simulink model "TS"  (R2024a)
settings: Solver=VariableStepAuto  StartTime=0.0  StopTime=10*10^-6  RelTol=1e-3
undefined symbols (not defined in the file): c1, c3
libraries: commblkcod2 x1, commofdm x1, commdigbbndam3 x1, commseqgen3 x1
settings Model: Creator=Honest  LastModifiedBy=NEYMAR
settings RTWCC: GPUComputeCapability=3.5

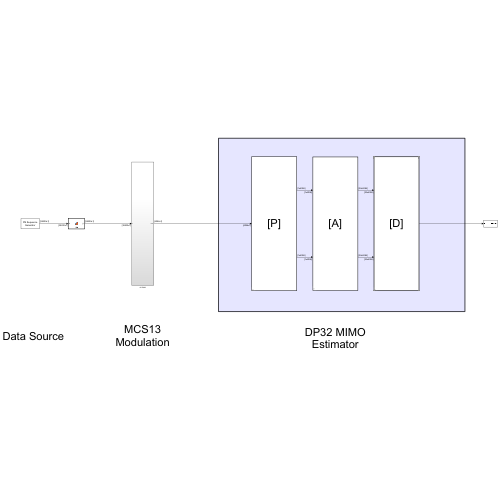
[thumbnail: Simulink's stored preview of the top-level diagram]
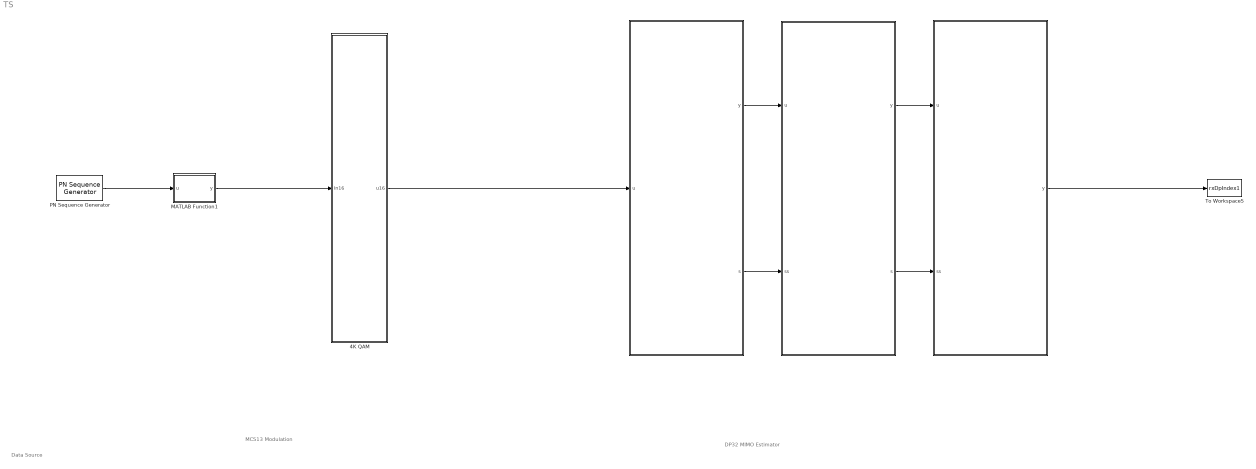
== system TS ==
  note: Data Source
  note: MCS13 Modulation
  note: DP32 MIMO Estimator
  " " : MATLAB Function  TreatAsAtomicUnit=on
  " " : MATLAB Function  TreatAsAtomicUnit=on
  "    " : MATLAB Function  TreatAsAtomicUnit=on
  4K QAM : Subsystem
  MATLAB Function1 : MATLAB Function  TreatAsAtomicUnit=on
  PN Sequence Generator : commseqgen3/PN Sequence Generator  poly='z^15 + z^14 + 1'  ini_sta=[0 0 0 0 0 0 0 0 0 0 0 0 0 0 1]  outBitMaskSource=Dialog parameter  shift=0  outVarSiz=off  maxOutSizeMode=Dialog parameter  maxOutSize=[10 1]  Ts=3.472222*10^-10  sampPerFrame=39200  reset=off  bitPackedOutputs=off  outDataType=double  numPackedBits=8  bitPackDataSigned=off  bitPackedOutDType=double
  To Workspace5 : ToWorkspace  VariableName=rxDpIndex1  SampleTime=-1
      settings: MaxDataPoints=1  Save2DSignal=2-D array (concatenate along first dimension)
  wires:
  4K QAM/1(u16) -> " "/1(u)
  PN Sequence Generator/1 -> MATLAB Function1/1(u)
  " "/1(y) -> "    "/1(u)
  "    "/1(y) -> " "/1(u)
  " "/1(y) -> To Workspace5/1
  " "/2(s) -> "    "/2(ss)
  "    "/2(s) -> " "/2(ss)
  MATLAB Function1/1(y) -> 4K QAM/1(In16)

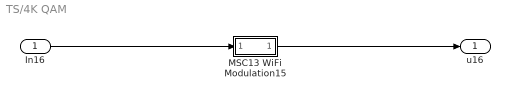
== system TS/4K QAM ==
  In16 : Inport
  MSC13 WiFi Modulation15 : Subsystem
  u16 : Outport
  wires:
  In16/1 -> MSC13 WiFi Modulation15/1(In1)
  MSC13 WiFi Modulation15/1(Out1) -> u16/1

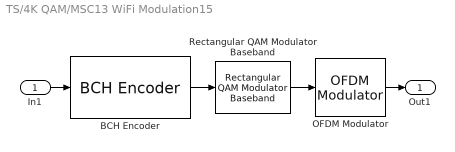
== system TS/4K QAM/MSC13 WiFi Modulation15 ==
  In1 : Inport
  BCH Encoder : commblkcod2/BCH Encoder  n=47040  k=39200  specShortening=off  shortenedK=5  specGenPoly=off  genPoly='X^10 + X^8 + X^5 + X^4 + X^2 + X + 1'  specPrimPoly=off  prPoly='X^4 + X + 1'  specDisableGenCheck=off  specPuncture=off  punctVec=[ones(8,1); zeros(2,1)]
  OFDM Modulator : commofdm/OFDM Modulator  StatePerturbationForJacobian=1.0e-05  FFTLength=4096  NumGuardBandCarriers=[88; 88]  InsertDCNull=off  PilotInputPort=off  PilotCarrierIndices=[52;104;156;208;260]  CyclicPrefixLength=0  Windowing=off  WindowLength=1  OversamplingFactor=1  NumSymbols=1  NumTransmitAntennas=1  SimulateUsing=Interpreted execution
  Rectangular QAM Modulator Baseband : commdigbbndam3/Rectangular QAM Modulator Baseband  M=4096  InType=Bit  Enc=Gray  Mapping=[0:15]  PowType=Min. distance between symbols  MinDist=2  AvgPow=1  PeakPow=1  Ph=0  outDtype=double  outWordLen=16  outUDDataType=sfix(16)  outFracLenMode=Best precision  outFracLen=15  outDataTypeStr=double  outLastDataTypeStr=double
  Out1 : Outport
  wires:
  Rectangular QAM Modulator Baseband/1 -> OFDM Modulator/1
  OFDM Modulator/1 -> Out1/1
  BCH Encoder/1 -> Rectangular QAM Modulator Baseband/1
  In1/1 -> BCH Encoder/1

== matlab function TS/MATLAB Function1 ==
  data: u input; y output
function y = fcn(u)

u(1:39200,1) = 1;

y = u;

== matlab function TS/  ==
  data: u input; y output; s output
function [y, s] = fcn(u)
    
        Walsh = [
            1	1	1	1	1	1	1	1	1	1	1	1	1	1	1	1	1	1	1	1	1	1	1	1	1	1	1	1	1	1	1	1;
																															    
            1	-1	1	-1	1	-1	1	-1	1	-1	1	-1	1	-1	1	-1	1	-1	1	-1	1	-1	1	-1	1	-1	1	-1	1	-1	1	-1;
																															            
            1	1	-1	-1	1	1	-1	-1	1	1	-1	-1	1	1	-1	-1	1	1	-1	-1	1	1	-1	-1	1	1	-1	-1	1	1	-1	-1;
																															            
            1	-1	-1	1	1	-1	-1	1	1	-1	-1	1	1	-1	-1	1	1	-1	-1	1	1	-1	-1	1	1	-1	-1	1	1	-1	-1	1;
																															            
            1	1	1	1	-1	-1	-1	-1	1	1	1	1	-1	-1	-1	-1	1	1	1	1	-1	-1	-1	-1	1	1	1	1	-1	-1	-1	-1;
																															            
            1	-1	1	-1	-1	1	-1	1	1	-1	1	-1	-1	1	-1	1	1	-1	1	-1	-1	1	-1	1	1	-1	1	-1	-1	1	-1	1;
																															            
            1	1	-1	-1	-1	-1	1	1	1	1	-1	-1	-1	-1	1	1	1	1	-1	-1	-1	-1	1	1	1	1	-1	-1	-1	-1	1	1;
																															            
            1	-1	-1	1	-1	1	1	-1	1	-1	-1	1	-1	1	1	-1	1	-1	-1	1	-1	1	1	-1	1	-1	-1	1	-1	1	1	-1;
																															            
            1	1	1	1	1	1	1	1	-1	-1	-1	-1	-1	-1	-1	-1	1	1	1	1	1	1	1	1	-1	-1	-1	-1	-1	-1	-1	-1;
																															            
            1	-1	1	-1	1	-1	1	-1	-1	1	-1	1	-1	1	-1	1	1	-1	1	-1	1	-1	1	-1	-1	1	-1	1	-1	1	-1	1;
																															            
            1	1	-1	-1	1	1	-1	-1	-1	-1	1	1	-1	-1	1	1	1	1	-1	-1	1	1	-1	-1	-1	-1	1	1	-1	-1	1	1;
																															            
            1	-1	-1	1	1	-1	-1	1	-1	1	1	-1	-1	1	1	-1	1	-1	-1	1	1	-1	-1	1	-1	1	1	-1	-1	1	1	-1;
																															            
            1	1	1	1	-1	-1	-1	-1	-1	-1	-1	-1	1	1	1	1	1	1	1	1	-1	-1	-1	-1	-1	-1	-1	-1	1	1	1	1;
																															            
            1	-1	1	-1	-1	1	-1	1	-1	1	-1	1	1	-1	1	-1	1	-1	1	-1	-1	1	-1	1	-1	1	-1	1	1	-1	1	-1;
																															            
            1	1	-1	-1	-1	-1	1	1	-1	-1	1	1	1	1	-1	-1	1	1	-1	-1	-1	-1	1	1	-1	-1	1	1	1	1	-1	-1;
																															            
            1	-1	-1	1	-1	1	1	-1	-1	1	1	-1	1	-1	-1	1	1	-1	-1	1	-1	1	1	-1	-1	1	1	-1	1	-1	-1	1;
																															            
            1	1	1	1	1	1	1	1	1	1	1	1	1	1	1	1	-1	-1	-1	-1	-1	-1	-1	-1	-1	-1	-1	-1	-1	-1	-1	-1;
																															            
            1	-1	1	-1	1	-1	1	-1	1	-1	1	-1	1	-1	1	-1	-1	1	-1	1	-1	1	-1	1	-1	1	-1	1	-1	1	-1	1;
																															            
            1	1	-1	-1	1	1	-1	-1	1	1	-1	-1	1	1	-1	-1	-1	-1	1	1	-1	-1	1	1	-1	-1	1	1	-1	-1	1	1;
																															            
            1	-1	-1	1	1	-1	-1	1	1	-1	-1	1	1	-1	-1	1	-1	1	1	-1	-1	1	1	-1	-1	1	1	-1	-1	1	1	-1;
																															            
            1	1	1	1	-1	-1	-1	-1	1	1	1	1	-1	-1	-1	-1	-1	-1	-1	-1	1	1	1	1	-1	-1	-1	-1	1	1	1	1;
																															            
            1	-1	1	-1	-1	1	-1	1	1	-1	1	-1	-1	1	-1	1	-1	1	-1	1	1	-1	1	-1	-1	1	-1	1	1	-1	1	-1;
																															            
            1	1	-1	-1	-1	-1	1	1	1	1	-1	-1	-1	-1	1	1	-1	-1	1	1	1	1	-1	-1	-1	-1	1	1	1	1	-1	-1;
																															            
            1	-1	-1	1	-1	1	1	-1	1	-1	-1	1	-1	1	1	-1	-1	1	1	-1	1	-1	-1	1	-1	1	1	-1	1	-1	-1	1;
																															            
            1	1	1	1	1	1	1	1	-1	-1	-1	-1	-1	-1	-1	-1	-1	-1	-1	-1	-1	-1	-1	-1	1	1	1	1	1	1	1	1;
																															            
            1	-1	1	-1	1	-1	1	-1	-1	1	-1	1	-1	1	-1	1	-1	1	-1	1	-1	1	-1	1	1	-1	1	-1	1	-1	1	-1;
																															            
            1	1	-1	-1	1	1	-1	-1	-1	-1	1	1	-1	-1	1	1	-1	-1	1	1	-1	-1	1	1	1	1	-1	-1	1	1	-1	-1;
																															            
            1	-1	-1	1	1	-1	-1	1	-1	1	1	-1	-1	1	1	-1	-1	1	1	-1	-1	1	1	-1	1	-1	-1	1	1	-1	-1	1;
																															            
            1	1	1	1	-1	-1	-1	-1	-1	-1	-1	-1	1	1	1	1	-1	-1	-1	-1	1	1	1	1	1	1	1	1	-1	-1	-1	-1;
																															            
            1	-1	1	-1	-1	1	-1	1	-1	1	-1	1	1	-1	1	-1	-1	1	-1	1	1	-1	1	-1	1	-1	1	-1	-1	1	-1	1;
																															            
            1	1	-1	-1	-1	-1	1	1	-1	-1	1	1	1	1	-1	-1	-1	-1	1	1	1	1	-1	-1	1	1	-1	-1	-1	-1	1	1;
																															            
            1	-1	-1	1	-1	1	1	-1	-1	1	1	-1	1	-1	-1	1	-1	1	1	-1	1	-1	-1	1	1	-1	-1	1	-1	1	1	-1;
        ];

        Increased_Walsh = Walsh(:, repelem(1:size(Walsh, 2), 16));
        
        Ext_Walsh = repmat(Increased_Walsh, [1, 8]);
        
        % 32 streams
        ProcessedInput = reshape(u,4096,1)';
        
        % Polarization
        Polarization = Ext_Walsh(1, :);
        assignin('base', "P", Polarization);

y = Polarization;
s = ProcessedInput;

== matlab function TS/     ==
  data: u input; y output; ss input; s output
function [y, s] = fcn(u, ss)

        % Aggregated polarization
        TempAggregatedPolarization = reshape(u', 1, []);
        TAPRowClone = repmat(TempAggregatedPolarization, 32, 1);
        assignin('base', 'PA', TAPRowClone);

        % Aggregated streams
        TempAggregatedProcessedInput = reshape(ss, 1, 4096);
        TAPIRowClone = repmat(TempAggregatedProcessedInput, 32, 1);
        
y = TAPRowClone;
s = TAPIRowClone;

== matlab function TS/  ==
  data: u input; y output; ss input; c1 parameter; c3 parameter
function y = fcn(u, ss, c1, c3)
        
        Walsh = [
            1	1	1	1	1	1	1	1	1	1	1	1	1	1	1	1	1	1	1	1	1	1	1	1	1	1	1	1	1	1	1	1;
																															    
            1	-1	1	-1	1	-1	1	-1	1	-1	1	-1	1	-1	1	-1	1	-1	1	-1	1	-1	1	-1	1	-1	1	-1	1	-1	1	-1;
																															            
            1	1	-1	-1	1	1	-1	-1	1	1	-1	-1	1	1	-1	-1	1	1	-1	-1	1	1	-1	-1	1	1	-1	-1	1	1	-1	-1;
																															            
            1	-1	-1	1	1	-1	-1	1	1	-1	-1	1	1	-1	-1	1	1	-1	-1	1	1	-1	-1	1	1	-1	-1	1	1	-1	-1	1;
																															            
            1	1	1	1	-1	-1	-1	-1	1	1	1	1	-1	-1	-1	-1	1	1	1	1	-1	-1	-1	-1	1	1	1	1	-1	-1	-1	-1;
																															            
            1	-1	1	-1	-1	1	-1	1	1	-1	1	-1	-1	1	-1	1	1	-1	1	-1	-1	1	-1	1	1	-1	1	-1	-1	1	-1	1;
																															            
            1	1	-1	-1	-1	-1	1	1	1	1	-1	-1	-1	-1	1	1	1	1	-1	-1	-1	-1	1	1	1	1	-1	-1	-1	-1	1	1;
																															            
            1	-1	-1	1	-1	1	1	-1	1	-1	-1	1	-1	1	1	-1	1	-1	-1	1	-1	1	1	-1	1	-1	-1	1	-1	1	1	-1;
																															            
            1	1	1	1	1	1	1	1	-1	-1	-1	-1	-1	-1	-1	-1	1	1	1	1	1	1	1	1	-1	-1	-1	-1	-1	-1	-1	-1;
																															            
            1	-1	1	-1	1	-1	1	-1	-1	1	-1	1	-1	1	-1	1	1	-1	1	-1	1	-1	1	-1	-1	1	-1	1	-1	1	-1	1;
																															            
            1	1	-1	-1	1	1	-1	-1	-1	-1	1	1	-1	-1	1	1	1	1	-1	-1	1	1	-1	-1	-1	-1	1	1	-1	-1	1	1;
																															            
            1	-1	-1	1	1	-1	-1	1	-1	1	1	-1	-1	1	1	-1	1	-1	-1	1	1	-1	-1	1	-1	1	1	-1	-1	1	1	-1;
																															            
            1	1	1	1	-1	-1	-1	-1	-1	-1	-1	-1	1	1	1	1	1	1	1	1	-1	-1	-1	-1	-1	-1	-1	-1	1	1	1	1;
																															            
            1	-1	1	-1	-1	1	-1	1	-1	1	-1	1	1	-1	1	-1	1	-1	1	-1	-1	1	-1	1	-1	1	-1	1	1	-1	1	-1;
																															            
            1	1	-1	-1	-1	-1	1	1	-1	-1	1	1	1	1	-1	-1	1	1	-1	-1	-1	-1	1	1	-1	-1	1	1	1	1	-1	-1;
																															            
            1	-1	-1	1	-1	1	1	-1	-1	1	1	-1	1	-1	-1	1	1	-1	-1	1	-1	1	1	-1	-1	1	1	-1	1	-1	-1	1;
																															            
            1	1	1	1	1	1	1	1	1	1	1	1	1	1	1	1	-1	-1	-1	-1	-1	-1	-1	-1	-1	-1	-1	-1	-1	-1	-1	-1;
																															            
            1	-1	1	-1	1	-1	1	-1	1	-1	1	-1	1	-1	1	-1	-1	1	-1	1	-1	1	-1	1	-1	1	-1	1	-1	1	-1	1;
																															            
            1	1	-1	-1	1	1	-1	-1	1	1	-1	-1	1	1	-1	-1	-1	-1	1	1	-1	-1	1	1	-1	-1	1	1	-1	-1	1	1;
																															            
            1	-1	-1	1	1	-1	-1	1	1	-1	-1	1	1	-1	-1	1	-1	1	1	-1	-1	1	1	-1	-1	1	1	-1	-1	1	1	-1;
																															            
            1	1	1	1	-1	-1	-1	-1	1	1	1	1	-1	-1	-1	-1	-1	-1	-1	-1	1	1	1	1	-1	-1	-1	-1	1	1	1	1;
																															            
            1	-1	1	-1	-1	1	-1	1	1	-1	1	-1	-1	1	-1	1	-1	1	-1	1	1	-1	1	-1	-1	1	-1	1	1	-1	1	-1;
																															            
            1	1	-1	-1	-1	-1	1	1	1	1	-1	-1	-1	-1	1	1	-1	-1	1	1	1	1	-1	-1	-1	-1	1	1	1	1	-1	-1;
																															            
            1	-1	-1	1	-1	1	1	-1	1	-1	-1	1	-1	1	1	-1	-1	1	1	-1	1	-1	-1	1	-1	1	1	-1	1	-1	-1	1;
																															            
            1	1	1	1	1	1	1	1	-1	-1	-1	-1	-1	-1	-1	-1	-1	-1	-1	-1	-1	-1	-1	-1	1	1	1	1	1	1	1	1;
																															            
            1	-1	1	-1	1	-1	1	-1	-1	1	-1	1	-1	1	-1	1	-1	1	-1	1	-1	1	-1	1	1	-1	1	-1	1	-1	1	-1;
																															            
            1	1	-1	-1	1	1	-1	-1	-1	-1	1	1	-1	-1	1	1	-1	-1	1	1	-1	-1	1	1	1	1	-1	-1	1	1	-1	-1;
																															            
            1	-1	-1	1	1	-1	-1	1	-1	1	1	-1	-1	1	1	-1	-1	1	1	-1	-1	1	1	-1	1	-1	-1	1	1	-1	-1	1;
																															            
            1	1	1	1	-1	-1	-1	-1	-1	-1	-1	-1	1	1	1	1	-1	-1	-1	-1	1	1	1	1	1	1	1	1	-1	-1	-1	-1;
																															            
            1	-1	1	-1	-1	1	-1	1	-1	1	-1	1	1	-1	1	-1	-1	1	-1	1	1	-1	1	-1	1	-1	1	-1	-1	1	-1	1;
																															            
            1	1	-1	-1	-1	-1	1	1	-1	-1	1	1	1	1	-1	-1	-1	-1	1	1	1	1	-1	-1	1	1	-1	-1	-1	-1	1	1;
																															            
            1	-1	-1	1	-1	1	1	-1	-1	1	1	-1	1	-1	-1	1	-1	1	1	-1	1	-1	-1	1	1	-1	-1	1	-1	1	1	-1;
        ];

        Increased_Walsh = Walsh(:, repelem(1:size(Walsh, 2), 16));
        
        Ext_Walsh = repmat(Increased_Walsh, [1, 8]);
        
        % Polarization to be multiplied to Receieved Polarization
        R_matrix = Ext_Walsh;
        
        % Multiplication of Polarization and Depolarization
        Result_matrix = u .* R_matrix;
        assignin('base', 'PAD', Result_matrix);
        
        % Sample by sample, Replace 1s with cos, -1s with sin
        % c1 is cos, c3 is sin
        for i = 1:32
            for j = 1:4096

                if Result_matrix(i, j) == 1
                    Result_matrix(i, j) = c1;
                else
                    Result_matrix(i, j) = c3;
                end            

            end
        end

        assignin('base', 'RM1', Result_matrix);
        
        SR_M = rand(32, 1);

        for i = 1:32
            for k = 1:1
                
                start_index = 4096 * (k-1) + 1;
                end_index = start_index + 4095;
                SR_M(i, k) = sum(Result_matrix(i, start_index:end_index))/4096;

            end
        end

        assignin('base', 'SRM', SR_M);

        SR_M = SR_M';

        ChDPI = SR_M(1);

        assignin('base', 'ChDPI', ChDPI);

        RxDPI = sum(SR_M(2:32))/31;

        %assignin('base', 'RxDPI', RxDPI);

        %assign the rxDpIndex into workspace

        assignin('base', "rxDpIndex1", RxDPI);
       
y = RxDPI;
